simulink model "Linear_model_LQR"  (R2025b)
settings: Solver=VariableStepAuto  StartTime=0.0  StopTime=10.0  RelTol=1e-3
values from neighbouring files (symbols this model uses):
  A1 = [0  1; 0  0]    [drone_model_parameters.mat]
  A2 = [0 0 0 0 0 0 9.81 0 1 0 0 0 ... (16 elements, 4x4)]    [drone_model_parameters.mat]
  A3 = [0 0 0 0 0 0 -9.81 0 1 0 0 0 ... (16 elements, 4x4)]    [drone_model_parameters.mat]
  A4 = [0  1; 0  0]    [drone_model_parameters.mat]
  B1 = [0 15.873015873]    [drone_model_parameters.mat]
  B2 = [0 0 0 17156.7786432]    [drone_model_parameters.mat]
  B3 = [0 0 0 13948.7522841]    [drone_model_parameters.mat]
  B4 = [0 33333.3333333]    [drone_model_parameters.mat]
  C1 = [1  0; 0  1]    [drone_model_parameters.mat]
  C2 = [1 0 0 0 0 1 0 0 0 0 1 0 ... (16 elements, 4x4)]    [drone_model_parameters.mat]
  C3 = [1 0 0 0 0 1 0 0 0 0 1 0 ... (16 elements, 4x4)]    [drone_model_parameters.mat]
  C4 = [1  0; 0  1]    [drone_model_parameters.mat]
  K1 = K1_lqr(1:2)    [Q13.m]    (also in drone_model_parameters.mat = [2.89638225196 1.1683082486]; full_lqr_simulink_run.m)
  K2 = K2_lqr(1:4)    [Q13.m]    (also in drone_model_parameters.mat = [3.01752211722 2.83921349975 1.28158254887 0.316750647665]; full_lqr_simulink_run.m)
  K3 = K3_lqr(1:4)    [Q13.m]    (also in drone_model_parameters.mat = [-3.01765609095 2.83974612226 -1.2817103927 0.316870901912]; full_lqr_simulink_run.m)
  K4 = K4_lqr(1:2)    [Q13.m]    (also in drone_model_parameters.mat = [1.73235075562 0.316392068556]; full_lqr_simulink_run.m)
  ki1 = -K1_lqr(3)    [Q13.m]    (also in drone_model_parameters.mat = 3.16227766017; full_lqr_simulink_run.m)
  ki2 = -K2_lqr(5)    [Q13.m]    (also in drone_model_parameters.mat = 3.16227766017; full_lqr_simulink_run.m)
  ki3 = -K3_lqr(5)    [Q13.m]    (also in drone_model_parameters.mat = -3.16227766017; full_lqr_simulink_run.m)
  ki4 = -K4_lqr(3)    [Q13.m]    (also in drone_model_parameters.mat = 3.16227766017; full_lqr_simulink_run.m)
  noise_P_lat = zeros(1,4)    [Q13.m]    (also in drone_model_parameters.mat = [0.009 0.003 0.002 1e-05]; full_lqr_simulink_run.m; noise_model_parameters.m = [var_P_r2,  var_P_th1, var_P_v2,  var_P_om1] * Ts)
  noise_P_lon = zeros(1,4)    [Q13.m]    (also in drone_model_parameters.mat = [0.009 0.002 0.002 1e-05]; full_lqr_simulink_run.m; noise_model_parameters.m = [var_P_r1,  var_P_th2, var_P_v1,  var_P_om2] * Ts)
  noise_P_vert = [0 0]    [Q13.m]    (also in drone_model_parameters.mat = [0.001 0.0001]; full_lqr_simulink_run.m; noise_model_parameters.m = [var_P_r3,  var_P_v3]  * Ts)
  noise_P_yaw = [0 0]    [Q13.m]    (also in drone_model_parameters.mat = [0.001 1e-05]; full_lqr_simulink_run.m; noise_model_parameters.m = [var_P_th3, var_P_om3] * Ts)
  phi_ref = 0    [Q13.m]    (also in drone_model_parameters.mat; full_lqr_simulink_run.m)
  Ts = 0.01    [Q13.m]    (also in drone_model_parameters.mat; full_lqr_simulink_run.m)
  x0_1 = [0; 0]    [Q13.m]    (also in drone_model_parameters.mat = [0 0]; full_lqr_simulink_run.m)
  x0_2 = [0; 0; 0; 0]    [Q13.m]    (also in drone_model_parameters.mat = [0 0 0 0]; full_lqr_simulink_run.m)
  x0_3 = [0; 0; 0; 0]    [Q13.m]    (also in drone_model_parameters.mat = [0 0 0 0]; full_lqr_simulink_run.m)
  x0_4 = [0; 0]    [Q13.m]    (also in drone_model_parameters.mat = [0 0]; full_lqr_simulink_run.m)
  x0_obs1 = [0 0]    [drone_model_parameters.mat]    (also in full_lqr_simulink_run.m = [0; 0])
  x0_obs2 = [0 0 0 0]    [drone_model_parameters.mat]    (also in full_lqr_simulink_run.m = [0; 0; 0; 0])
  x0_obs3 = [0 0 0 0]    [drone_model_parameters.mat]    (also in full_lqr_simulink_run.m = [0; 0; 0; 0])
  x0_obs4 = [0 0]    [drone_model_parameters.mat]    (also in full_lqr_simulink_run.m = [0; 0])
  x_ref = 4    [Q13.m]    (also in drone_model_parameters.mat; full_lqr_simulink_run.m)
  z_ref = 4    [Q13.m]    (also in drone_model_parameters.mat; full_lqr_simulink_run.m)
undefined symbols (not defined in the file or in its folder): L1, L2, L3, L4
libraries: simulink x8
settings Model: Creator=joaom  LastModifiedBy=joaom
settings DataIOCC: SaveFormat=Array

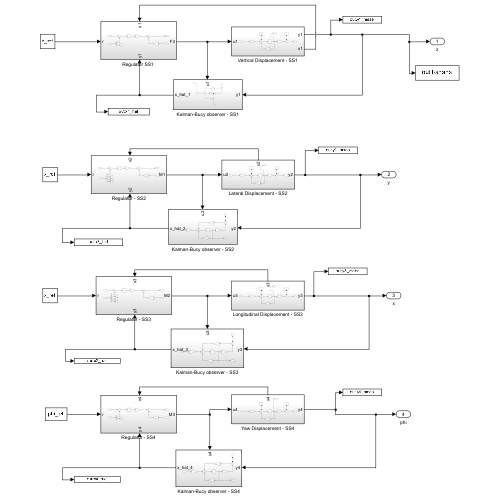
[thumbnail: Simulink's stored preview of the top-level diagram]
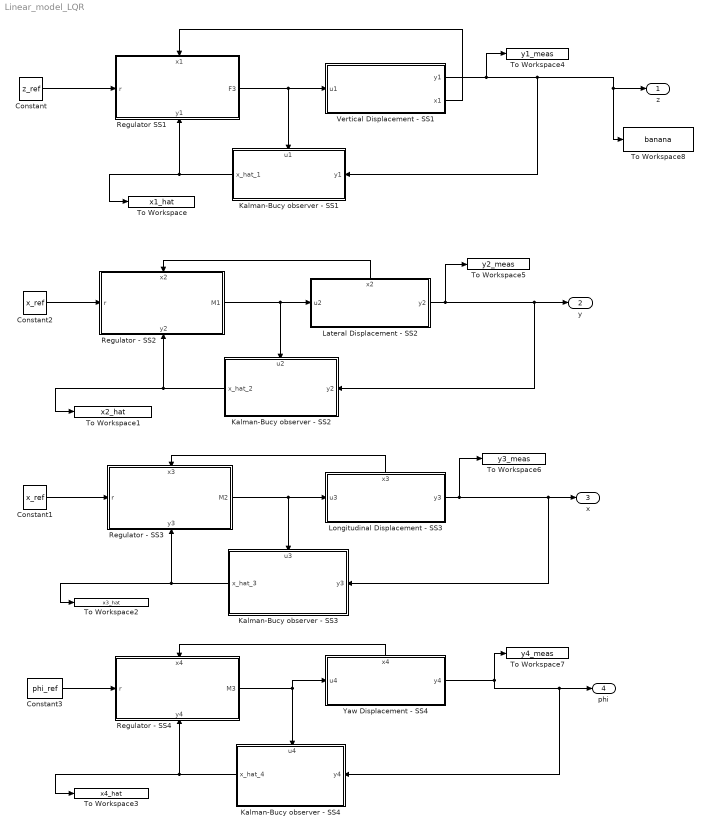
== system Linear_model_LQR ==
  Constant : Constant  Value=z_ref
  Constant1 : Constant  Value=x_ref
  Constant2 : Constant  Value=x_ref
  Constant3 : Constant  Value=phi_ref
  Kalman-Bucy observer - SS1 : Subsystem
      settings: PortSchema="{\"entries\":[{\"content\":{\"sides\":[{\"content\":{\"connectorIds\":[\"Out1\"]},\"type\":\"ConnectorPlacement.EquallySpacedRectSide\",\"uuid\":\"3a34d9e3-ef6b-4e0e-ad1c-a8e9abb9cb50\"},{\"content\":{\"connectorIds\":[\"In2\"],\"side\":\"RIGHT\"},\"type\":\"ConnectorPlacement.EquallySpacedRectSide\",\"uuid\":\"1b685036-9c62-4d8c-a792-6e44f47fda20\"},{\"content\":{\"connectorIds\":[\"In1\"],\"side\":\"TOP\"},\"type\":\"ConnectorPlacement.EquallySpacedRectSide\",\"uuid\":\"5c00f917-5739-44a5-95b0-e7bd6f61a97f\"}]},\"type\":\"ConnectorPlacement.EquallySpacedConnector\",\"uuid\":\"e365f2b2-c96f-4048-9751-de98e4d7538e\"}],\"packageUris\":[\"http://schema.mathworks.com/mf0/Connector/R2020b\"],\"version\":\"1.0\"}"
  Kalman-Bucy observer - SS2 : Subsystem
      settings: PortSchema="{\"entries\":[{\"content\":{\"sides\":[{\"content\":{\"connectorIds\":[\"Out1\"]},\"type\":\"ConnectorPlacement.EquallySpacedRectSide\",\"uuid\":\"3a34d9e3-ef6b-4e0e-ad1c-a8e9abb9cb50\"},{\"content\":{\"connectorIds\":[\"In2\"],\"side\":\"RIGHT\"},\"type\":\"ConnectorPlacement.EquallySpacedRectSide\",\"uuid\":\"1b685036-9c62-4d8c-a792-6e44f47fda20\"},{\"content\":{\"connectorIds\":[\"In1\"],\"side\":\"TOP\"},\"type\":\"ConnectorPlacement.EquallySpacedRectSide\",\"uuid\":\"5c00f917-5739-44a5-95b0-e7bd6f61a97f\"}]},\"type\":\"ConnectorPlacement.EquallySpacedConnector\",\"uuid\":\"e365f2b2-c96f-4048-9751-de98e4d7538e\"}],\"packageUris\":[\"http://schema.mathworks.com/mf0/Connector/R2020b\"],\"version\":\"1.0\"}"
  Kalman-Bucy observer - SS3 : Subsystem
      settings: PortSchema="{\"entries\":[{\"content\":{\"sides\":[{\"content\":{\"connectorIds\":[\"Out1\"]},\"type\":\"ConnectorPlacement.EquallySpacedRectSide\",\"uuid\":\"3a34d9e3-ef6b-4e0e-ad1c-a8e9abb9cb50\"},{\"content\":{\"connectorIds\":[\"In2\"],\"side\":\"RIGHT\"},\"type\":\"ConnectorPlacement.EquallySpacedRectSide\",\"uuid\":\"1b685036-9c62-4d8c-a792-6e44f47fda20\"},{\"content\":{\"connectorIds\":[\"In1\"],\"side\":\"TOP\"},\"type\":\"ConnectorPlacement.EquallySpacedRectSide\",\"uuid\":\"5c00f917-5739-44a5-95b0-e7bd6f61a97f\"}]},\"type\":\"ConnectorPlacement.EquallySpacedConnector\",\"uuid\":\"e365f2b2-c96f-4048-9751-de98e4d7538e\"}],\"packageUris\":[\"http://schema.mathworks.com/mf0/Connector/R2020b\"],\"version\":\"1.0\"}"
  Kalman-Bucy observer - SS4 : Subsystem
      settings: PortSchema="{\"entries\":[{\"content\":{\"sides\":[{\"content\":{\"connectorIds\":[\"Out1\"]},\"type\":\"ConnectorPlacement.EquallySpacedRectSide\",\"uuid\":\"3a34d9e3-ef6b-4e0e-ad1c-a8e9abb9cb50\"},{\"content\":{\"connectorIds\":[\"In2\"],\"side\":\"RIGHT\"},\"type\":\"ConnectorPlacement.EquallySpacedRectSide\",\"uuid\":\"1b685036-9c62-4d8c-a792-6e44f47fda20\"},{\"content\":{\"connectorIds\":[\"In1\"],\"side\":\"TOP\"},\"type\":\"ConnectorPlacement.EquallySpacedRectSide\",\"uuid\":\"5c00f917-5739-44a5-95b0-e7bd6f61a97f\"}]},\"type\":\"ConnectorPlacement.EquallySpacedConnector\",\"uuid\":\"e365f2b2-c96f-4048-9751-de98e4d7538e\"}],\"packageUris\":[\"http://schema.mathworks.com/mf0/Connector/R2020b\"],\"version\":\"1.0\"}"
  Lateral Displacement - SS2 : Subsystem
      settings: PortSchema="{\"entries\":[{\"content\":{\"sides\":[{\"content\":{\"connectorIds\":[\"In1\"]},\"type\":\"ConnectorPlacement.EquallySpacedRectSide\",\"uuid\":\"000fe622-0d2e-408f-a9fc-e5e03571fbc5\"},{\"content\":{\"connectorIds\":[\"Out1\"],\"side\":\"RIGHT\"},\"type\":\"ConnectorPlacement.EquallySpacedRectSide\",\"uuid\":\"78fe74da-3ec5-4952-a234-4a11e91b7a96\"},{\"content\":{\"connectorIds\":[\"Out2\"],\"side\":\"TOP\"},\"type\":\"ConnectorPlacement.EquallySpacedRectSide\",\"uuid\":\"aafedc52-0c51-42cc-bd8f-17c6bb8e3ea7\"}]},\"type\":\"ConnectorPlacement.EquallySpacedConnector\",\"uuid\":\"c23ce463-d1b8-4aee-9748-091893bc77a5\"}],\"packageUris\":[\"http://schema.mathworks.com/mf0/Connector/R2020b\"],\"version\":\"1.0\"}"
  Longitudinal Displacement - SS3 : Subsystem
      settings: PortSchema="{\"entries\":[{\"content\":{\"sides\":[{\"content\":{\"connectorIds\":[\"In1\"]},\"type\":\"ConnectorPlacement.EquallySpacedRectSide\",\"uuid\":\"000fe622-0d2e-408f-a9fc-e5e03571fbc5\"},{\"content\":{\"connectorIds\":[\"Out1\"],\"side\":\"RIGHT\"},\"type\":\"ConnectorPlacement.EquallySpacedRectSide\",\"uuid\":\"78fe74da-3ec5-4952-a234-4a11e91b7a96\"},{\"content\":{\"connectorIds\":[\"Out2\"],\"side\":\"TOP\"},\"type\":\"ConnectorPlacement.EquallySpacedRectSide\",\"uuid\":\"aafedc52-0c51-42cc-bd8f-17c6bb8e3ea7\"}]},\"type\":\"ConnectorPlacement.EquallySpacedConnector\",\"uuid\":\"c23ce463-d1b8-4aee-9748-091893bc77a5\"}],\"packageUris\":[\"http://schema.mathworks.com/mf0/Connector/R2020b\"],\"version\":\"1.0\"}"
  Regulator - SS2 : Subsystem
      settings: PortSchema="{\"entries\":[{\"content\":{\"sides\":[{\"content\":{\"connectorIds\":[\"In1\"]},\"type\":\"ConnectorPlacement.EquallySpacedRectSide\",\"uuid\":\"88111a94-f44e-4900-bd50-8e0aad39585f\"},{\"content\":{\"connectorIds\":[\"Out1\"],\"side\":\"RIGHT\"},\"type\":\"ConnectorPlacement.EquallySpacedRectSide\",\"uuid\":\"5258e968-599c-4ea3-bcfe-6bc79328b7b7\"},{\"content\":{\"connectorIds\":[\"In2\"],\"side\":\"TOP\"},\"type\":\"ConnectorPlacement.EquallySpacedRectSide\",\"uuid\":\"a4dacb5f-a91b-4773-b391-8d6e0b4fd6cf\"},{\"content\":{\"connectorIds\":[\"In3\"],\"side\":\"BOTTOM\"},\"type\":\"ConnectorPlacement.EquallySpacedRectSide\",\"uuid\":\"e2351862-dfcc-4d34-9606-068d4022ef4e\"}]},\"type\":\"ConnectorPlacement.EquallySpacedConnector\",\"uuid\":\"9200008f-efe3-4b90-8bfe-764cc35a5d3b\"}],\"packageUris\":[\"http://schema.mathworks.com/mf0/Connector/R2020b\"],\"version\":\"1.0\"}"
  Regulator - SS3 : Subsystem
      settings: PortSchema="{\"entries\":[{\"content\":{\"sides\":[{\"content\":{\"connectorIds\":[\"In1\"]},\"type\":\"ConnectorPlacement.EquallySpacedRectSide\",\"uuid\":\"88111a94-f44e-4900-bd50-8e0aad39585f\"},{\"content\":{\"connectorIds\":[\"Out1\"],\"side\":\"RIGHT\"},\"type\":\"ConnectorPlacement.EquallySpacedRectSide\",\"uuid\":\"5258e968-599c-4ea3-bcfe-6bc79328b7b7\"},{\"content\":{\"connectorIds\":[\"In2\"],\"side\":\"TOP\"},\"type\":\"ConnectorPlacement.EquallySpacedRectSide\",\"uuid\":\"a4dacb5f-a91b-4773-b391-8d6e0b4fd6cf\"},{\"content\":{\"connectorIds\":[\"In3\"],\"side\":\"BOTTOM\"},\"type\":\"ConnectorPlacement.EquallySpacedRectSide\",\"uuid\":\"85ab8a27-52ad-4ccd-acf0-0ca2b6406dd1\"}]},\"type\":\"ConnectorPlacement.EquallySpacedConnector\",\"uuid\":\"9200008f-efe3-4b90-8bfe-764cc35a5d3b\"}],\"packageUris\":[\"http://schema.mathworks.com/mf0/Connector/R2020b\"],\"version\":\"1.0\"}"
  Regulator - SS4 : Subsystem
      settings: PortSchema="{\"entries\":[{\"content\":{\"sides\":[{\"content\":{\"connectorIds\":[\"In1\"]},\"type\":\"ConnectorPlacement.EquallySpacedRectSide\",\"uuid\":\"88111a94-f44e-4900-bd50-8e0aad39585f\"},{\"content\":{\"connectorIds\":[\"Out1\"],\"side\":\"RIGHT\"},\"type\":\"ConnectorPlacement.EquallySpacedRectSide\",\"uuid\":\"5258e968-599c-4ea3-bcfe-6bc79328b7b7\"},{\"content\":{\"connectorIds\":[\"In2\"],\"side\":\"TOP\"},\"type\":\"ConnectorPlacement.EquallySpacedRectSide\",\"uuid\":\"a4dacb5f-a91b-4773-b391-8d6e0b4fd6cf\"},{\"content\":{\"connectorIds\":[\"In3\"],\"side\":\"BOTTOM\"},\"type\":\"ConnectorPlacement.EquallySpacedRectSide\",\"uuid\":\"b2d28f28-1888-41cd-96eb-2b979c16ad18\"}]},\"type\":\"ConnectorPlacement.EquallySpacedConnector\",\"uuid\":\"9200008f-efe3-4b90-8bfe-764cc35a5d3b\"}],\"packageUris\":[\"http://schema.mathworks.com/mf0/Connector/R2020b\"],\"version\":\"1.0\"}"
  "Regulator SS1 " : Subsystem
      settings: PortSchema="{\"entries\":[{\"content\":{\"sides\":[{\"content\":{\"connectorIds\":[\"In1\"]},\"type\":\"ConnectorPlacement.EquallySpacedRectSide\",\"uuid\":\"b3654a7f-5063-48c0-9b36-91e0db63b0ba\"},{\"content\":{\"connectorIds\":[\"Out1\"],\"side\":\"RIGHT\"},\"type\":\"ConnectorPlacement.EquallySpacedRectSide\",\"uuid\":\"218488d6-68f2-41aa-8299-f3fb09ba40d8\"},{\"content\":{\"connectorIds\":[\"In2\"],\"side\":\"TOP\"},\"type\":\"ConnectorPlacement.EquallySpacedRectSide\",\"uuid\":\"ffca8f5f-99ce-4cfe-b848-505d5918397a\"},{\"content\":{\"connectorIds\":[\"In3\"],\"side\":\"BOTTOM\"},\"type\":\"ConnectorPlacement.EquallySpacedRectSide\",\"uuid\":\"0ee1b0b7-fa1d-4d2f-b721-1db90edeb8b7\"}]},\"type\":\"ConnectorPlacement.EquallySpacedConnector\",\"uuid\":\"97e1b17e-acc2-4e54-bcf8-8316abbe6834\"}],\"packageUris\":[\"http://schema.mathworks.com/mf0/Connector/R2020b\"],\"version\":\"1.0\"}"
  To Workspace : ToWorkspace  VariableName=x1_hat  SampleTime=-1
  To Workspace1 : ToWorkspace  VariableName=x2_hat  SampleTime=-1
  To Workspace2 : ToWorkspace  VariableName=x3_hat  SampleTime=-1
  To Workspace3 : ToWorkspace  VariableName=x4_hat  SampleTime=-1
  To Workspace4 : ToWorkspace  VariableName=y1_meas  SampleTime=-1
  To Workspace5 : ToWorkspace  VariableName=y2_meas  SampleTime=-1
  To Workspace6 : ToWorkspace  VariableName=y3_meas  SampleTime=-1
  To Workspace7 : ToWorkspace  VariableName=y4_meas  SampleTime=-1
  To Workspace8 : ToWorkspace  VariableName=banana  SaveFormat=Timeseries  SampleTime=-1
  Vertical Displacement - SS1 : Subsystem
  Yaw Displacement - SS4 : Subsystem
      settings: PortSchema="{\"entries\":[{\"content\":{\"sides\":[{\"content\":{\"connectorIds\":[\"In1\"]},\"type\":\"ConnectorPlacement.EquallySpacedRectSide\",\"uuid\":\"000fe622-0d2e-408f-a9fc-e5e03571fbc5\"},{\"content\":{\"connectorIds\":[\"Out1\"],\"side\":\"RIGHT\"},\"type\":\"ConnectorPlacement.EquallySpacedRectSide\",\"uuid\":\"78fe74da-3ec5-4952-a234-4a11e91b7a96\"},{\"content\":{\"connectorIds\":[\"Out2\"],\"side\":\"TOP\"},\"type\":\"ConnectorPlacement.EquallySpacedRectSide\",\"uuid\":\"aafedc52-0c51-42cc-bd8f-17c6bb8e3ea7\"}]},\"type\":\"ConnectorPlacement.EquallySpacedConnector\",\"uuid\":\"c23ce463-d1b8-4aee-9748-091893bc77a5\"}],\"packageUris\":[\"http://schema.mathworks.com/mf0/Connector/R2020b\"],\"version\":\"1.0\"}"
  z : Outport
  y : Outport  Port=2
  x : Outport  Port=3
  phi : Outport  Port=4
  wires:
  Constant/1 -> "Regulator SS1 "/1(r)
  "Regulator SS1 "/1(F3) -> Kalman-Bucy observer - SS1/1(u1), Vertical Displacement - SS1/1(u1)
  Regulator - SS2/1(M1) -> Kalman-Bucy observer - SS2/1(u2), Lateral Displacement - SS2/1(u2)
  Constant1/1 -> Regulator - SS3/1(r)
  Regulator - SS3/1(M2) -> Longitudinal Displacement - SS3/1(u3), Kalman-Bucy observer - SS3/1(u3)
  Yaw Displacement - SS4/1(y4) -> To Workspace7/1, Kalman-Bucy observer - SS4/2(y4), phi/1
  Constant3/1 -> Regulator - SS4/1(r)
  Regulator - SS4/1(M3) -> Kalman-Bucy observer - SS4/1(u4), Yaw Displacement - SS4/1(u4)
  Kalman-Bucy observer - SS3/1(x_hat_3) -> To Workspace2/1, Regulator - SS3/3(y3)
  Kalman-Bucy observer - SS4/1(x_hat_4) -> To Workspace3/1, Regulator - SS4/3(y4)
  Kalman-Bucy observer - SS2/1(x_hat_2) -> To Workspace1/1, Regulator - SS2/3(y2)
  Vertical Displacement - SS1/1(y1) -> Kalman-Bucy observer - SS1/2(y1), To Workspace8/1, z/1, To Workspace4/1
  Lateral Displacement - SS2/1(y2) -> To Workspace5/1, Kalman-Bucy observer - SS2/2(y2), y/1
  Longitudinal Displacement - SS3/1(y3) -> To Workspace6/1, Kalman-Bucy observer - SS3/2(y3), x/1
  Vertical Displacement - SS1/2(x1) -> "Regulator SS1 "/2(x1)
  Constant2/1 -> Regulator - SS2/1(r)
  Lateral Displacement - SS2/2(x2) -> Regulator - SS2/2(x2)
  Longitudinal Displacement - SS3/2(x3) -> Regulator - SS3/2(x3)
  Yaw Displacement - SS4/2(x4) -> Regulator - SS4/2(x4)
  Kalman-Bucy observer - SS1/1(x_hat_1) -> To Workspace/1, "Regulator SS1 "/3(y1)

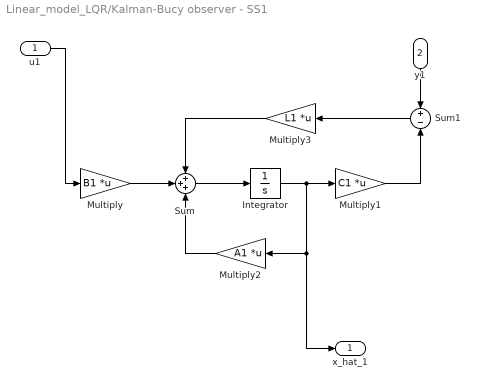
== system Linear_model_LQR/Kalman-Bucy observer - SS1 ==
  u1 : Inport
  y1 : Inport  Port=2
  Integrator : Integrator  InitialCondition=x0_obs1
  Multiply : Gain  Gain=B1  Multiplication=Matrix(K*u)
  Multiply1 : Gain  Gain=C1  Multiplication=Matrix(K*u)
  Multiply2 : Gain  Gain=A1  Multiplication=Matrix(K*u)
  Multiply3 : Gain  Gain=L1  Multiplication=Matrix(K*u)
  Sum : Sum  Inputs=+++
  Sum1 : Sum  Inputs=+|-
  x_hat_1 : Outport
  wires:
  Multiply2/1 -> Sum/3
  Sum/1 -> Integrator/1
  Integrator/1 -> x_hat_1/1, Multiply2/1, Multiply1/1
  u1/1 -> Multiply/1
  Multiply3/1 -> Sum/1
  Multiply/1 -> Sum/2
  Multiply1/1 -> Sum1/2
  y1/1 -> Sum1/1
  Sum1/1 -> Multiply3/1

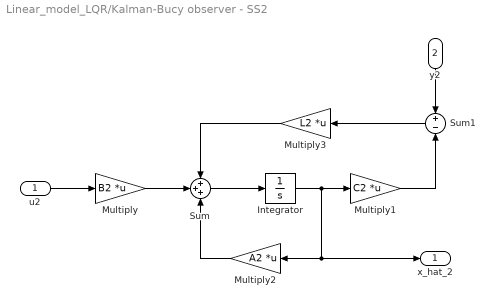
== system Linear_model_LQR/Kalman-Bucy observer - SS2 ==
  u2 : Inport
  y2 : Inport  Port=2
  Integrator : Integrator  InitialCondition=x0_obs2
  Multiply : Gain  Gain=B2  Multiplication=Matrix(K*u)
  Multiply1 : Gain  Gain=C2  Multiplication=Matrix(K*u)
  Multiply2 : Gain  Gain=A2  Multiplication=Matrix(K*u)
  Multiply3 : Gain  Gain=L2  Multiplication=Matrix(K*u)
  Sum : Sum  Inputs=+++
  Sum1 : Sum  Inputs=+|-
  x_hat_2 : Outport
  wires:
  Multiply2/1 -> Sum/3
  Sum/1 -> Integrator/1
  Integrator/1 -> x_hat_2/1, Multiply2/1, Multiply1/1
  u2/1 -> Multiply/1
  Multiply3/1 -> Sum/1
  Multiply/1 -> Sum/2
  Multiply1/1 -> Sum1/2
  y2/1 -> Sum1/1
  Sum1/1 -> Multiply3/1

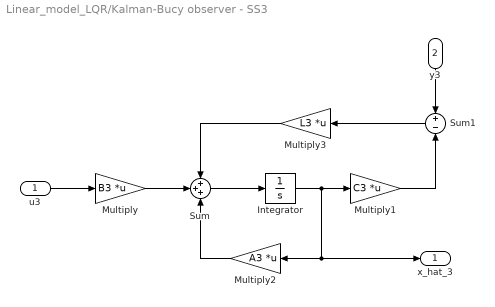
== system Linear_model_LQR/Kalman-Bucy observer - SS3 ==
  u3 : Inport
  y3 : Inport  Port=2
  Integrator : Integrator  InitialCondition=x0_obs3
  Multiply : Gain  Gain=B3  Multiplication=Matrix(K*u)
  Multiply1 : Gain  Gain=C3  Multiplication=Matrix(K*u)
  Multiply2 : Gain  Gain=A3  Multiplication=Matrix(K*u)
  Multiply3 : Gain  Gain=L3  Multiplication=Matrix(K*u)
  Sum : Sum  Inputs=+++
  Sum1 : Sum  Inputs=+|-
  x_hat_3 : Outport
  wires:
  Multiply2/1 -> Sum/3
  Sum/1 -> Integrator/1
  Integrator/1 -> x_hat_3/1, Multiply2/1, Multiply1/1
  u3/1 -> Multiply/1
  Multiply3/1 -> Sum/1
  Multiply/1 -> Sum/2
  Multiply1/1 -> Sum1/2
  y3/1 -> Sum1/1
  Sum1/1 -> Multiply3/1

== system Linear_model_LQR/Kalman-Bucy observer - SS4 ==
  u4 : Inport
  y4 : Inport  Port=2
  Integrator : Integrator  InitialCondition=x0_obs4
  Multiply : Gain  Gain=B4  Multiplication=Matrix(K*u)
  Multiply1 : Gain  Gain=C4  Multiplication=Matrix(K*u)
  Multiply2 : Gain  Gain=A4  Multiplication=Matrix(K*u)
  Multiply3 : Gain  Gain=L4  Multiplication=Matrix(K*u)
  Sum : Sum  Inputs=+++
  Sum1 : Sum  Inputs=+|-
  x_hat_4 : Outport
  wires:
  Multiply2/1 -> Sum/3
  Sum/1 -> Integrator/1
  Integrator/1 -> x_hat_4/1, Multiply2/1, Multiply1/1
  u4/1 -> Multiply/1
  Multiply3/1 -> Sum/1
  Multiply/1 -> Sum/2
  Multiply1/1 -> Sum1/2
  y4/1 -> Sum1/1
  Sum1/1 -> Multiply3/1

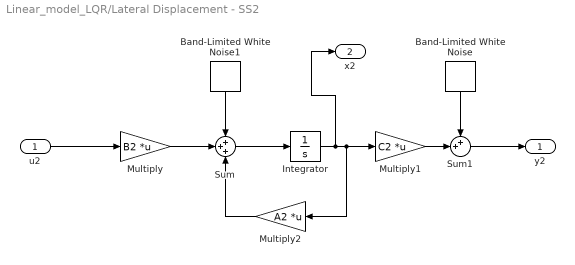
== system Linear_model_LQR/Lateral Displacement - SS2 ==
  u2 : Inport
  Band-Limited White Noise : simulink/Sources/Band-Limited White Noise  Cov=noise_M_lat  Ts=0.01  seed=[50 51 52 53]
  Band-Limited White Noise1 : simulink/Sources/Band-Limited White Noise  Cov=[noise_P_lat]  Ts=0.01  seed=[46 47 48 49]
  Integrator : Integrator  InitialCondition=x0_2
  Multiply : Gain  Gain=B2  Multiplication=Matrix(K*u)
  Multiply1 : Gain  Gain=C2  Multiplication=Matrix(K*u)
  Multiply2 : Gain  Gain=A2  Multiplication=Matrix(K*u)
  Sum : Sum  Inputs=+++
  Sum1 : Sum  Inputs=++|
  y2 : Outport
  x2 : Outport  Port=2
  wires:
  u2/1 -> Multiply/1
  Multiply/1 -> Sum/2
  Sum/1 -> Integrator/1
  Integrator/1 -> x2/1, Multiply2/1, Multiply1/1
  Multiply1/1 -> Sum1/2
  Sum1/1 -> y2/1
  Multiply2/1 -> Sum/3
  Band-Limited White Noise/1 -> Sum1/1
  Band-Limited White Noise1/1 -> Sum/1

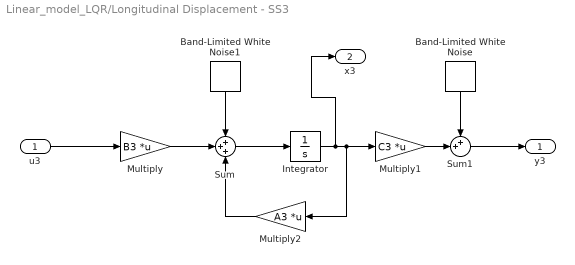
== system Linear_model_LQR/Longitudinal Displacement - SS3 ==
  u3 : Inport
  Band-Limited White Noise : simulink/Sources/Band-Limited White Noise  Cov=noise_M_lon  Ts=0.01  seed=[58 59 60 61]
  Band-Limited White Noise1 : simulink/Sources/Band-Limited White Noise  Cov=[noise_P_lon]  Ts=0.01  seed=[54 55 56 57]
  Integrator : Integrator  InitialCondition=x0_3
  Multiply : Gain  Gain=B3  Multiplication=Matrix(K*u)
  Multiply1 : Gain  Gain=C3  Multiplication=Matrix(K*u)
  Multiply2 : Gain  Gain=A3  Multiplication=Matrix(K*u)
  Sum : Sum  Inputs=+++
  Sum1 : Sum  Inputs=++|
  y3 : Outport
  x3 : Outport  Port=2
  wires:
  u3/1 -> Multiply/1
  Multiply/1 -> Sum/2
  Sum/1 -> Integrator/1
  Integrator/1 -> x3/1, Multiply2/1, Multiply1/1
  Multiply1/1 -> Sum1/2
  Sum1/1 -> y3/1
  Multiply2/1 -> Sum/3
  Band-Limited White Noise/1 -> Sum1/1
  Band-Limited White Noise1/1 -> Sum/1

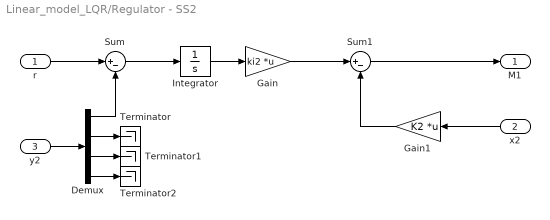
== system Linear_model_LQR/Regulator - SS2 ==
  r : Inport
  x2 : Inport  Port=2
  y2 : Inport  Port=3
  Demux : Demux
  Gain : Gain  Gain=ki2  Multiplication=Matrix(K*u)
  Gain1 : Gain  Gain=K2  Multiplication=Matrix(K*u)
  Integrator : Integrator
  Sum : Sum  Inputs=|+-
  Sum1 : Sum  Inputs=|+-
  Terminator : Terminator
  Terminator1 : Terminator
  Terminator2 : Terminator
  M1 : Outport
  wires:
  x2/1 -> Gain1/1
  Gain/1 -> Sum1/1
  Demux/2 -> Terminator/1
  Demux/3 -> Terminator1/1
  Sum1/1 -> M1/1
  Gain1/1 -> Sum1/2
  Sum/1 -> Integrator/1
  y2/1 -> Demux/1
  Integrator/1 -> Gain/1
  Demux/1 -> Sum/2
  Demux/4 -> Terminator2/1
  r/1 -> Sum/1

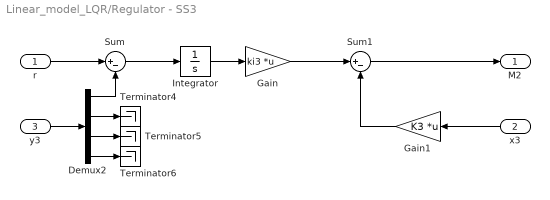
== system Linear_model_LQR/Regulator - SS3 ==
  r : Inport
  x3 : Inport  Port=2
  y3 : Inport  Port=3
  Demux2 : Demux
  Gain : Gain  Gain=ki3  Multiplication=Matrix(K*u)
  Gain1 : Gain  Gain=K3  Multiplication=Matrix(K*u)
  Integrator : Integrator
  Sum : Sum  Inputs=|+-
  Sum1 : Sum  Inputs=|+-
  Terminator4 : Terminator
  Terminator5 : Terminator
  Terminator6 : Terminator
  M2 : Outport
  wires:
  Gain1/1 -> Sum1/2
  Sum1/1 -> M2/1
  Demux2/4 -> Terminator6/1
  r/1 -> Sum/1
  Demux2/2 -> Terminator4/1
  Demux2/1 -> Sum/2
  Demux2/3 -> Terminator5/1
  y3/1 -> Demux2/1
  Sum/1 -> Integrator/1
  x3/1 -> Gain1/1
  Gain/1 -> Sum1/1
  Integrator/1 -> Gain/1

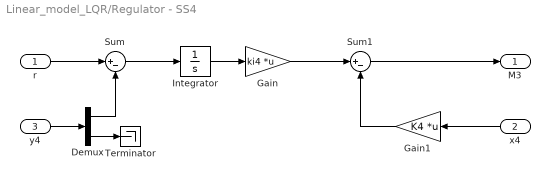
== system Linear_model_LQR/Regulator - SS4 ==
  r : Inport
  x4 : Inport  Port=2
  y4 : Inport  Port=3
  Demux : Demux  Outputs=2
  Gain : Gain  Gain=ki4  Multiplication=Matrix(K*u)
  Gain1 : Gain  Gain=K4  Multiplication=Matrix(K*u)
  Integrator : Integrator
  Sum : Sum  Inputs=|+-
  Sum1 : Sum  Inputs=|+-
  Terminator : Terminator
  M3 : Outport
  wires:
  Gain1/1 -> Sum1/2
  Sum/1 -> Integrator/1
  Sum1/1 -> M3/1
  r/1 -> Sum/1
  y4/1 -> Demux/1
  Integrator/1 -> Gain/1
  Demux/1 -> Sum/2
  Gain/1 -> Sum1/1
  x4/1 -> Gain1/1
  Demux/2 -> Terminator/1

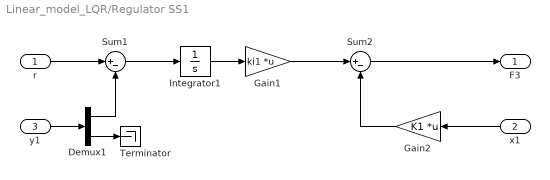
== system Linear_model_LQR/Regulator SS1  ==
  r : Inport
  x1 : Inport  Port=2
  y1 : Inport  Port=3
  Demux1 : Demux  Outputs=2
  Gain1 : Gain  Gain=ki1  Multiplication=Matrix(K*u)
  Gain2 : Gain  Gain=K1  Multiplication=Matrix(K*u)
  Integrator1 : Integrator
  Sum1 : Sum  Inputs=|+-
  Sum2 : Sum  Inputs=|+-
  Terminator : Terminator
  F3 : Outport
  wires:
  Demux1/1 -> Sum1/2
  Integrator1/1 -> Gain1/1
  x1/1 -> Gain2/1
  r/1 -> Sum1/1
  Gain1/1 -> Sum2/1
  Gain2/1 -> Sum2/2
  y1/1 -> Demux1/1
  Sum2/1 -> F3/1
  Sum1/1 -> Integrator1/1
  Demux1/2 -> Terminator/1

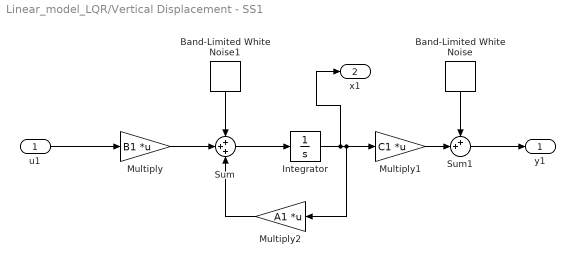
== system Linear_model_LQR/Vertical Displacement - SS1 ==
  u1 : Inport
  Band-Limited White Noise : simulink/Sources/Band-Limited White Noise  Cov=noise_M_vert  Ts=0.01  seed=[44 45]
  Band-Limited White Noise1 : simulink/Sources/Band-Limited White Noise  Cov=[noise_P_vert]  Ts=Ts  seed=[42 43]
  Integrator : Integrator  InitialCondition=x0_1
  Multiply : Gain  Gain=B1  Multiplication=Matrix(K*u)
  Multiply1 : Gain  Gain=C1  Multiplication=Matrix(K*u)
  Multiply2 : Gain  Gain=A1  Multiplication=Matrix(K*u)
  Sum : Sum  Inputs=+++
  Sum1 : Sum  Inputs=++|
  y1 : Outport
  x1 : Outport  Port=2
  wires:
  u1/1 -> Multiply/1
  Multiply/1 -> Sum/2
  Sum/1 -> Integrator/1
  Integrator/1 -> x1/1, Multiply2/1, Multiply1/1
  Multiply1/1 -> Sum1/2
  Sum1/1 -> y1/1
  Multiply2/1 -> Sum/3
  Band-Limited White Noise/1 -> Sum1/1
  Band-Limited White Noise1/1 -> Sum/1

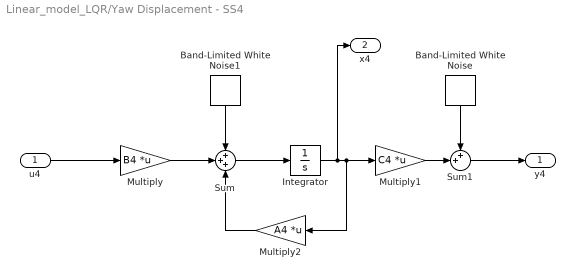
== system Linear_model_LQR/Yaw Displacement - SS4 ==
  u4 : Inport
  Band-Limited White Noise : simulink/Sources/Band-Limited White Noise  Cov=noise_M_yaw  Ts=0.01  seed=[64 65]
  Band-Limited White Noise1 : simulink/Sources/Band-Limited White Noise  Cov=[noise_P_yaw]  Ts=0.01  seed=[62 63]
  Integrator : Integrator  InitialCondition=x0_4
  Multiply : Gain  Gain=B4  Multiplication=Matrix(K*u)
  Multiply1 : Gain  Gain=C4  Multiplication=Matrix(K*u)
  Multiply2 : Gain  Gain=A4  Multiplication=Matrix(K*u)
  Sum : Sum  Inputs=+++
  Sum1 : Sum  Inputs=++|
  y4 : Outport
  x4 : Outport  Port=2
  wires:
  u4/1 -> Multiply/1
  Multiply/1 -> Sum/2
  Sum/1 -> Integrator/1
  Integrator/1 -> x4/1, Multiply2/1, Multiply1/1
  Multiply1/1 -> Sum1/2
  Sum1/1 -> y4/1
  Multiply2/1 -> Sum/3
  Band-Limited White Noise/1 -> Sum1/1
  Band-Limited White Noise1/1 -> Sum/1
